simulink model "simulacionModeloNoLinealTaoTaur"  (R2021a)
settings: Solver=VariableStepAuto  StartTime=0.0  StopTime=100  RelTol=1e-3
settings Model: Creator=jmata  LastModifiedBy=jmata

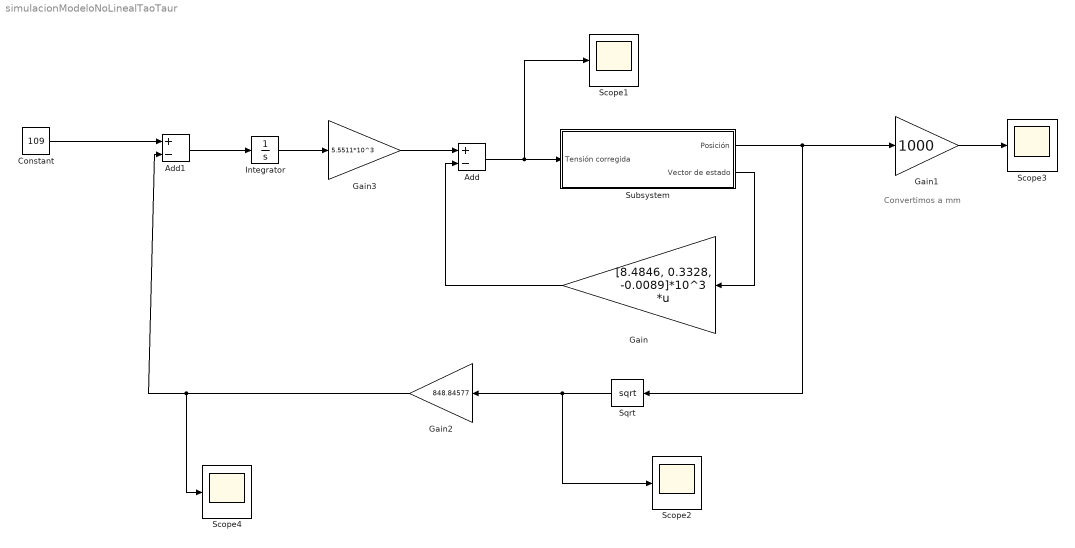
== system simulacionModeloNoLinealTaoTaur ==
  note: Convertimos a mm
  Add : Sum  Inputs=+-
  Add1 : Sum  Inputs=+-
  Constant : Constant  Value=109
  Gain : Gain  Gain=[8.4846, 0.3328, -0.0089]*10^3  Multiplication=Matrix(K*u)
  Gain1 : Gain  Gain=1000
  Gain2 : Gain  Gain=848.84577
  Gain3 : Gain  Gain=5.5511*10^3
  Integrator : Integrator
  Scope{1..4} (4 alike) : Scope
  Sqrt : Sqrt  SaturateOnIntegerOverflow=on
  Subsystem : Subsystem
  wires:
  Add/1 -> Scope1/1, Subsystem/1(Tensión corregida)
  Subsystem/2(Vector de estado) -> Gain/1
  Gain/1 -> Add/2
  Subsystem/1(Posición) -> Gain1/1, Sqrt/1
  Sqrt/1 -> Scope2/1, Gain2/1
  Gain2/1 -> Scope4/1, Add1/2
  Add1/1 -> Integrator/1
  Integrator/1 -> Gain3/1
  Gain3/1 -> Add/1
  Constant/1 -> Add1/1
  Gain1/1 -> Scope3/1

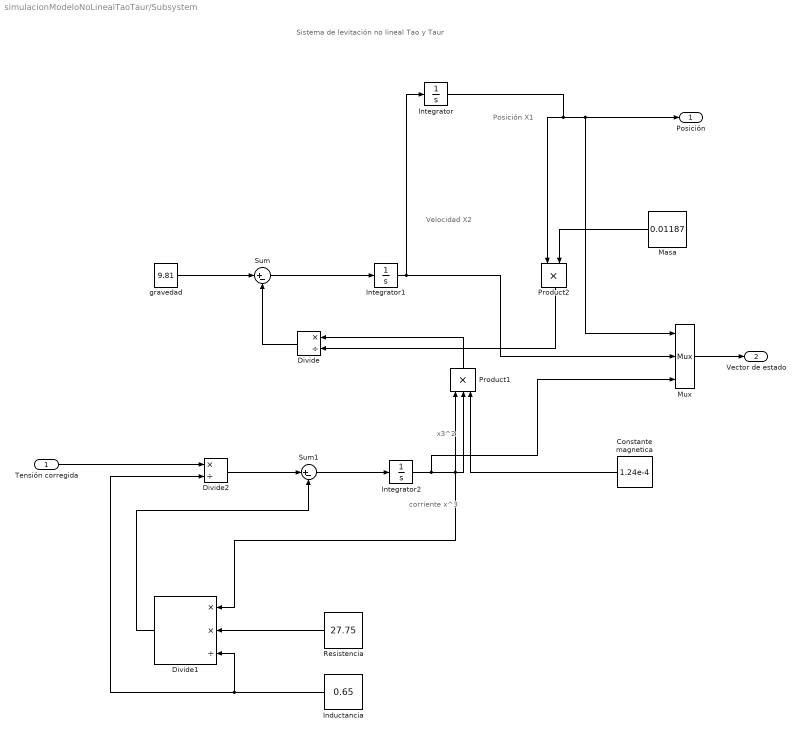
== system simulacionModeloNoLinealTaoTaur/Subsystem ==
  note: corriente x^3
  note: x3^2
  note: Velocidad X2
  note: Posición X1
  note: Sistema de levitación no lineal Tao y Taur
  Tensión corregida : Inport
  Constante magnetica : Constant  Value=1.24e-4
  Divide : Product  Inputs=*/
  Divide1 : Product  Inputs=**/
  Divide2 : Product  Inputs=*/
  Inductancia : Constant  Value=0.65
  Integrator : Integrator  InitialCondition=0.01612
  Integrator1 : Integrator
  Integrator2 : Integrator
  Masa : Constant  Value=0.01187
  Mux : Mux  Inputs=3
  Product1 : Product  Inputs=3
  Product2 : Product
  Resistencia : Constant  Value=27.75
  Sum : Sum  Inputs=|+-
  Sum1 : Sum  Inputs=|+-
  gravedad : Constant  Value=9.81
  Posición : Outport
  Vector de estado : Outport  Port=2
  wires:
  Integrator/1 -> Mux/1, Posición/1, Product2/1
  Integrator1/1 -> Mux/2, Integrator/1
  gravedad/1 -> Sum/1
  Divide/1 -> Sum/2
  Sum/1 -> Integrator1/1
  Integrator2/1 -> Mux/3, Divide1/1, Product1/1, Product1/2
  Constante magnetica/1 -> Product1/3
  Masa/1 -> Product2/2
  Product1/1 -> Divide/1
  Product2/1 -> Divide/2
  Inductancia/1 -> Divide2/2, Divide1/3
  Resistencia/1 -> Divide1/2
  Divide1/1 -> Sum1/2
  Sum1/1 -> Integrator2/1
  Tensión corregida/1 -> Divide2/1
  Divide2/1 -> Sum1/1
  Mux/1 -> Vector de estado/1
